simulink model "dynamic_QL"  (R2020b)
settings: Solver=VariableStepAuto  StartTime=0.0  StopTime=30.0  RelTol=1e-3
undefined symbols (not defined in the file or in its folder): loc, objects
libraries: mobileRoboticsLib x16, pid_lib x10
settings Model: Creator=Roozbeh  LastModifiedBy=Roozbeh

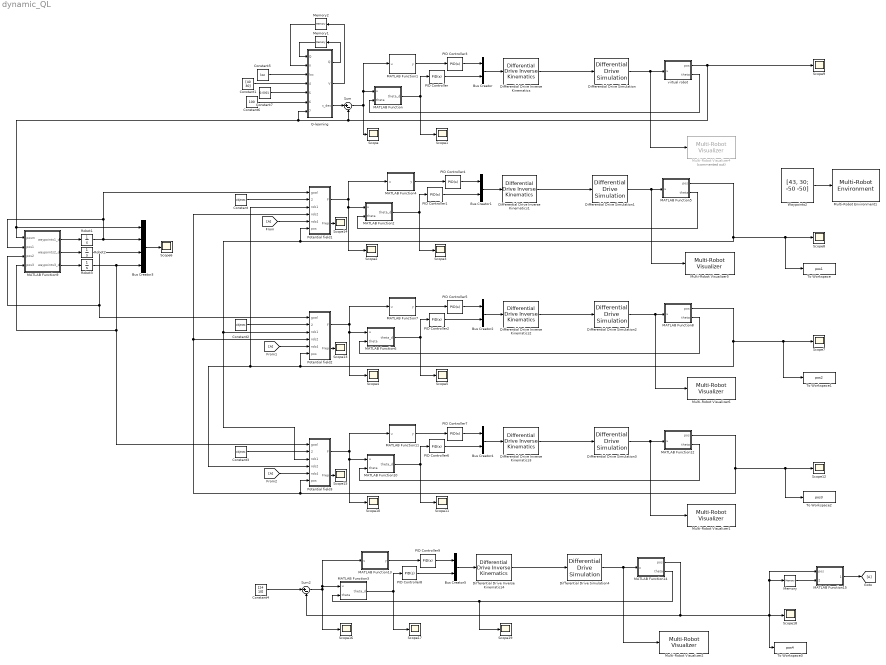
== system dynamic_QL ==
  Bus Creator{,1..2,4..5} (5 alike) : BusCreator  Inputs=2
  Bus Creator3 : BusCreator  Inputs=4
  Constant : Constant  Value=objects
  Constant1 : Constant  Value=[40 30]
  Constant2 : Constant  Value=objects
  Constant3 : Constant  Value=objects
  Constant4 : Constant  Value=[24 10]
  Constant5 : Constant  Value=loc
  Constant6 : Constant  Value=100
  Constant7 : Constant  Value=0.0001
  Differential Drive Inverse Kinematics{,1..4} (5 alike) : mobileRoboticsLib/Kinematic Models/Differential Drive/Differential Drive Inverse Kinematics  wheelRadius=0.1  wheelBase=0.5
      settings: SourceProductName=Mobile Robotics Simulation Toolbox
  Differential Drive Simulation : mobileRoboticsLib/Kinematic Models/Differential Drive/Differential Drive Simulation  wheelRadius=0.1  wheelBase=0.5  initX=6  initY=6  initAngle=0  Ts=0.05
      settings: SourceProductName=Mobile Robotics Simulation Toolbox
  Differential Drive Simulation1 : mobileRoboticsLib/Kinematic Models/Differential Drive/Differential Drive Simulation  wheelRadius=0.1  wheelBase=0.5  initX=8  initY=8  initAngle=0  Ts=0.05
      settings: SourceProductName=Mobile Robotics Simulation Toolbox
  Differential Drive Simulation2 : mobileRoboticsLib/Kinematic Models/Differential Drive/Differential Drive Simulation  wheelRadius=0.1  wheelBase=0.5  initX=4  initY=4  initAngle=0  Ts=0.05
      settings: SourceProductName=Mobile Robotics Simulation Toolbox
  Differential Drive Simulation3 : mobileRoboticsLib/Kinematic Models/Differential Drive/Differential Drive Simulation  wheelRadius=0.1  wheelBase=0.5  initX=4  initY=12  initAngle=0  Ts=0.05
      settings: SourceProductName=Mobile Robotics Simulation Toolbox
  Differential Drive Simulation4 : mobileRoboticsLib/Kinematic Models/Differential Drive/Differential Drive Simulation  wheelRadius=0.1  wheelBase=0.5  initX=24  initY=38  initAngle=0  Ts=0.05
      settings: SourceProductName=Mobile Robotics Simulation Toolbox
  MATLAB Function : MATLAB Function  TreatAsAtomicUnit=on
  MATLAB Function1 : MATLAB Function  TreatAsAtomicUnit=on
  MATLAB Function10 : MATLAB Function  TreatAsAtomicUnit=on
  MATLAB Function11 : MATLAB Function  TreatAsAtomicUnit=on
  MATLAB Function12 : MATLAB Function  TreatAsAtomicUnit=on
  MATLAB Function13 : MATLAB Function  TreatAsAtomicUnit=on
  MATLAB Function14 : MATLAB Function  TreatAsAtomicUnit=on
  MATLAB Function15 : MATLAB Function  TreatAsAtomicUnit=on
  MATLAB Function2 : MATLAB Function  TreatAsAtomicUnit=on
  MATLAB Function3 : MATLAB Function  TreatAsAtomicUnit=on
  MATLAB Function4 : MATLAB Function  TreatAsAtomicUnit=on
  MATLAB Function5 : MATLAB Function  TreatAsAtomicUnit=on
  MATLAB Function6 : MATLAB Function  TreatAsAtomicUnit=on
  MATLAB Function7 : MATLAB Function  TreatAsAtomicUnit=on
  MATLAB Function8 : MATLAB Function  TreatAsAtomicUnit=on
  MATLAB Function9 : MATLAB Function  TreatAsAtomicUnit=on
  Memory : Memory
  Memory1 : Memory  InitialCondition=zeros(size(loc,1) * size(loc,2), 8)
  Memory2 : Memory  InitialCondition=zeros(size(loc,1), size(loc,2))
  Multi-Robot Environment1 : mobileRoboticsLib/Environments/Multi-Robot Environment  numRobots=4  mapName=mapRooz  showWaypoints=on  showObjects=off  objectColors=[ 1, 0, 0; 0, 1, 0; 0, 0, 1 ]  objectMarkers='s'  showRobotIds=on  plotSensorLines=on
      settings: SourceProductName=Mobile Robotics Simulation Toolbox
  Multi-Robot Visualizer1 : mobileRoboticsLib/Environments/Multi-Robot Visualizer  idx=3  radius=0.5  robotColor=[0 0 1]  showTraj=off  hasLidar=off  sensorOffset=[0,0]  scanAngles=[-pi/4 0 pi/4]  maxNumScans=0  hasObjDetector=off  objDetectorOffset=[0,0]  objDetectorAngle=0  objDetectorFOV=pi/3  objDetectorMaxRange=5  hasRobotDetector=off  robotDetectorOffset=[0,0]  robotDetectorAngle=0  robotDetectorFOV=pi/3  robotDetectorMaxRange=5  robotDetectorNumDetections=0
      settings: SourceProductName=Mobile Robotics Simulation Toolbox
  Multi-Robot Visualizer2 : mobileRoboticsLib/Environments/Multi-Robot Visualizer  idx=4  radius=0.5  robotColor=[0 0 0]  showTraj=off  hasLidar=off  sensorOffset=[0,0]  scanAngles=[-pi/4 0 pi/4]  maxNumScans=0  hasObjDetector=off  objDetectorOffset=[0,0]  objDetectorAngle=0  objDetectorFOV=pi/3  objDetectorMaxRange=5  hasRobotDetector=off  robotDetectorOffset=[0,0]  robotDetectorAngle=0  robotDetectorFOV=pi/3  robotDetectorMaxRange=5  robotDetectorNumDetections=0
      settings: SourceProductName=Mobile Robotics Simulation Toolbox
  Multi-Robot Visualizer4 : mobileRoboticsLib/Environments/Multi-Robot Visualizer  Commented=on  idx=1  radius=0.5  robotColor=[0 0 1]  showTraj=off  hasLidar=off  sensorOffset=[0,0]  scanAngles=[-pi/4 0 pi/4]  maxNumScans=0  hasObjDetector=off  objDetectorOffset=[0,0]  objDetectorAngle=0  objDetectorFOV=pi/3  objDetectorMaxRange=5  hasRobotDetector=off  robotDetectorOffset=[0,0]  robotDetectorAngle=0  robotDetectorFOV=pi/3  robotDetectorMaxRange=5  robotDetectorNumDetections=0
      settings: SourceProductName=Mobile Robotics Simulation Toolbox
  Multi-Robot Visualizer5 : mobileRoboticsLib/Environments/Multi-Robot Visualizer  idx=1  radius=0.5  robotColor=[0 1 0]  showTraj=off  hasLidar=off  sensorOffset=[0,0]  scanAngles=[-pi/4 0 pi/4]  maxNumScans=0  hasObjDetector=off  objDetectorOffset=[0,0]  objDetectorAngle=0  objDetectorFOV=pi/3  objDetectorMaxRange=5  hasRobotDetector=off  robotDetectorOffset=[0,0]  robotDetectorAngle=0  robotDetectorFOV=pi/3  robotDetectorMaxRange=5  robotDetectorNumDetections=0
      settings: SourceProductName=Mobile Robotics Simulation Toolbox
  Multi-Robot Visualizer6 : mobileRoboticsLib/Environments/Multi-Robot Visualizer  idx=2  radius=0.5  robotColor=[1 0 0]  showTraj=off  hasLidar=off  sensorOffset=[0,0]  scanAngles=[-pi/4 0 pi/4]  maxNumScans=0  hasObjDetector=off  objDetectorOffset=[0,0]  objDetectorAngle=0  objDetectorFOV=pi/3  objDetectorMaxRange=5  hasRobotDetector=off  robotDetectorOffset=[0,0]  robotDetectorAngle=0  robotDetectorFOV=pi/3  robotDetectorMaxRange=5  robotDetectorNumDetections=0
      settings: SourceProductName=Mobile Robotics Simulation Toolbox
  PID Controller : pid_lib/PID Controller  Controller=PID  Form=Parallel  TimeDomain=Continuous-time  UseExternalTs=off  SampleTime=-1  IntegratorMethod=Forward Euler  FilterMethod=Forward Euler  ControllerParametersSource=internal  P=10  I=1  D=0  UseFilter=on  N=100  TunerSelectOption=Transfer Function Based (PID Tuner App)  InitialConditionSource=internal  InitialConditionForIntegrator=0  InitialConditionForFilter=0  DifferentiatorICPrevScaledInput=0  ExternalReset=none  TrackingMode=off  Kt=1  LimitOutput=off  SatLimitsSource=internal  UpperSaturationLimit=3  LowerSaturationLimit=-3  LinearizeAsGain=on  AntiWindupMode=none  Kb=1  POutMin=[]  POutMax=[]  IOutMin=[]  IOutMax=[]  DOutMin=[]  DOutMax=[]  NOutMin=[]  NOutMax=[]  SumOutMin=[]  SumOutMax=[]  SaturationOutMin=[]  SaturationOutMax=[]  PParamMin=[]  PParamMax=[]  IParamMin=[]  IParamMax=[]  DParamMin=[]  DParamMax=[]  NParamMin=[]  NParamMax=[]  KbParamMin=[]  KbParamMax=[]  KtParamMin=[]  KtParamMax=[]  KbOutMin=[]  KbOutMax=[]  KtOutMin=[]  KtOutMax=[]  IntegratorOutMin=[]  IntegratorOutMax=[]  FilterOutMin=[]  FilterOutMax=[]  SumI1OutMin=[]  SumI1OutMax=[]  SumI2OutMin=[]  SumI2OutMax=[]  SumI3OutMin=[]  SumI3OutMax=[]  SumI4OutMin=[]  SumI4OutMax=[]  SumDOutMin=[]  SumDOutMax=[]  DifferentiatorOutMin=[]  DifferentiatorOutMax=[]  FilterDiffOutCoefMin=[]  FilterDiffOutCoefMax=[]  ReciprocalOutMin=[]  ReciprocalOutMax=[]  SumDenOutMin=[]  SumDenOutMax=[]  SumNumOutMin=[]  SumNumOutMax=[]  DivideOutMin=[]  DivideOutMax=[]  UdiffTsProdOutMin=[]  UdiffTsProdOutMax=[]  NTsProdOutMin=[]  NTsProdOutMax=[]  UintegralTsProdOutMin=[]  UintegralTsProdOutMax=[]  UngainTsProdOutMin=[]  UngainTsProdOutMax=[]  IntegratorContinuousStateAttributes=''  IntegratorStateMustResolveToSignalObject=off  IntegratorRTWStateStorageClass=Auto  FilterContinuousStateAttributes=''  FilterStateMustResolveToSignalObject=off  FilterRTWStateStorageClass=Auto  ParallelPVariant=InternalParameters  IdealPVariant=Disabled  IVariant=InternalParameters  DVariant=InternalParameters  IntegratorVariant=Continuous  SatVariant=Disabled  AWVariant=Passthrough  PCopyVariant=Disabled  TRVariant=Disabled  FdbkBlocksVariant=Forward  IdealPFdbkVariant=Disabled  SatFdbkVariant=Disabled  DerivativeFilterVariant=ContFilter  NVariant=InternalParameters  NCopyVariant=Disabled  FilterICVariant=InternalICsFilter  IntegratorICVariant=InternalICs  ExternalResetVariant=Disabled  TRSumVariant=Passthrough  SumFdbkVariant=Disabled  SumVariant=Sum_PID  TsampFilterVariant=InternalTs  TsampNgainVariant=Passthrough  TsampIntegralVariant=Passthrough  ExternalSaturationOutDataTypeStr=Inherit: Same as second input
  PID Controller1 : pid_lib/PID Controller  Controller=PID  Form=Parallel  TimeDomain=Continuous-time  UseExternalTs=off  SampleTime=-1  IntegratorMethod=Forward Euler  FilterMethod=Forward Euler  ControllerParametersSource=internal  P=10  I=1  D=0  UseFilter=on  N=100  TunerSelectOption=Transfer Function Based (PID Tuner App)  InitialConditionSource=internal  InitialConditionForIntegrator=0  InitialConditionForFilter=0  DifferentiatorICPrevScaledInput=0  ExternalReset=none  TrackingMode=off  Kt=1  LimitOutput=on  SatLimitsSource=internal  UpperSaturationLimit=10  LowerSaturationLimit=-10  LinearizeAsGain=on  AntiWindupMode=none  Kb=1  POutMin=[]  POutMax=[]  IOutMin=[]  IOutMax=[]  DOutMin=[]  DOutMax=[]  NOutMin=[]  NOutMax=[]  SumOutMin=[]  SumOutMax=[]  SaturationOutMin=[]  SaturationOutMax=[]  PParamMin=[]  PParamMax=[]  IParamMin=[]  IParamMax=[]  DParamMin=[]  DParamMax=[]  NParamMin=[]  NParamMax=[]  KbParamMin=[]  KbParamMax=[]  KtParamMin=[]  KtParamMax=[]  KbOutMin=[]  KbOutMax=[]  KtOutMin=[]  KtOutMax=[]  IntegratorOutMin=[]  IntegratorOutMax=[]  FilterOutMin=[]  FilterOutMax=[]  SumI1OutMin=[]  SumI1OutMax=[]  SumI2OutMin=[]  SumI2OutMax=[]  SumI3OutMin=[]  SumI3OutMax=[]  SumI4OutMin=[]  SumI4OutMax=[]  SumDOutMin=[]  SumDOutMax=[]  DifferentiatorOutMin=[]  DifferentiatorOutMax=[]  FilterDiffOutCoefMin=[]  FilterDiffOutCoefMax=[]  ReciprocalOutMin=[]  ReciprocalOutMax=[]  SumDenOutMin=[]  SumDenOutMax=[]  SumNumOutMin=[]  SumNumOutMax=[]  DivideOutMin=[]  DivideOutMax=[]  UdiffTsProdOutMin=[]  UdiffTsProdOutMax=[]  NTsProdOutMin=[]  NTsProdOutMax=[]  UintegralTsProdOutMin=[]  UintegralTsProdOutMax=[]  UngainTsProdOutMin=[]  UngainTsProdOutMax=[]  IntegratorContinuousStateAttributes=''  IntegratorStateMustResolveToSignalObject=off  IntegratorRTWStateStorageClass=Auto  FilterContinuousStateAttributes=''  FilterStateMustResolveToSignalObject=off  FilterRTWStateStorageClass=Auto  ParallelPVariant=InternalParameters  IdealPVariant=Disabled  IVariant=InternalParameters  DVariant=InternalParameters  IntegratorVariant=Continuous  SatVariant=Enabled  AWVariant=Passthrough  PCopyVariant=Disabled  TRVariant=Disabled  FdbkBlocksVariant=Forward  IdealPFdbkVariant=Disabled  SatFdbkVariant=Disabled  DerivativeFilterVariant=ContFilter  NVariant=InternalParameters  NCopyVariant=Disabled  FilterICVariant=InternalICsFilter  IntegratorICVariant=InternalICs  ExternalResetVariant=Disabled  TRSumVariant=Passthrough  SumFdbkVariant=Disabled  SumVariant=Sum_PID  TsampFilterVariant=InternalTs  TsampNgainVariant=Passthrough  TsampIntegralVariant=Passthrough  ExternalSaturationOutDataTypeStr=Inherit: Same as second input
  PID Controller2 : pid_lib/PID Controller  Controller=PID  Form=Parallel  TimeDomain=Continuous-time  UseExternalTs=off  SampleTime=-1  IntegratorMethod=Forward Euler  FilterMethod=Forward Euler  ControllerParametersSource=internal  P=10  I=1  D=0  UseFilter=on  N=100  TunerSelectOption=Transfer Function Based (PID Tuner App)  InitialConditionSource=internal  InitialConditionForIntegrator=0  InitialConditionForFilter=0  DifferentiatorICPrevScaledInput=0  ExternalReset=none  TrackingMode=off  Kt=1  LimitOutput=on  SatLimitsSource=internal  UpperSaturationLimit=10  LowerSaturationLimit=-10  LinearizeAsGain=on  AntiWindupMode=none  Kb=1  POutMin=[]  POutMax=[]  IOutMin=[]  IOutMax=[]  DOutMin=[]  DOutMax=[]  NOutMin=[]  NOutMax=[]  SumOutMin=[]  SumOutMax=[]  SaturationOutMin=[]  SaturationOutMax=[]  PParamMin=[]  PParamMax=[]  IParamMin=[]  IParamMax=[]  DParamMin=[]  DParamMax=[]  NParamMin=[]  NParamMax=[]  KbParamMin=[]  KbParamMax=[]  KtParamMin=[]  KtParamMax=[]  KbOutMin=[]  KbOutMax=[]  KtOutMin=[]  KtOutMax=[]  IntegratorOutMin=[]  IntegratorOutMax=[]  FilterOutMin=[]  FilterOutMax=[]  SumI1OutMin=[]  SumI1OutMax=[]  SumI2OutMin=[]  SumI2OutMax=[]  SumI3OutMin=[]  SumI3OutMax=[]  SumI4OutMin=[]  SumI4OutMax=[]  SumDOutMin=[]  SumDOutMax=[]  DifferentiatorOutMin=[]  DifferentiatorOutMax=[]  FilterDiffOutCoefMin=[]  FilterDiffOutCoefMax=[]  ReciprocalOutMin=[]  ReciprocalOutMax=[]  SumDenOutMin=[]  SumDenOutMax=[]  SumNumOutMin=[]  SumNumOutMax=[]  DivideOutMin=[]  DivideOutMax=[]  UdiffTsProdOutMin=[]  UdiffTsProdOutMax=[]  NTsProdOutMin=[]  NTsProdOutMax=[]  UintegralTsProdOutMin=[]  UintegralTsProdOutMax=[]  UngainTsProdOutMin=[]  UngainTsProdOutMax=[]  IntegratorContinuousStateAttributes=''  IntegratorStateMustResolveToSignalObject=off  IntegratorRTWStateStorageClass=Auto  FilterContinuousStateAttributes=''  FilterStateMustResolveToSignalObject=off  FilterRTWStateStorageClass=Auto  ParallelPVariant=InternalParameters  IdealPVariant=Disabled  IVariant=InternalParameters  DVariant=InternalParameters  IntegratorVariant=Continuous  SatVariant=Enabled  AWVariant=Passthrough  PCopyVariant=Disabled  TRVariant=Disabled  FdbkBlocksVariant=Forward  IdealPFdbkVariant=Disabled  SatFdbkVariant=Disabled  DerivativeFilterVariant=ContFilter  NVariant=InternalParameters  NCopyVariant=Disabled  FilterICVariant=InternalICsFilter  IntegratorICVariant=InternalICs  ExternalResetVariant=Disabled  TRSumVariant=Passthrough  SumFdbkVariant=Disabled  SumVariant=Sum_PID  TsampFilterVariant=InternalTs  TsampNgainVariant=Passthrough  TsampIntegralVariant=Passthrough  ExternalSaturationOutDataTypeStr=Inherit: Same as second input
  PID Controller3 : pid_lib/PID Controller  Controller=PID  Form=Parallel  TimeDomain=Continuous-time  UseExternalTs=off  SampleTime=-1  IntegratorMethod=Forward Euler  FilterMethod=Forward Euler  ControllerParametersSource=internal  P=5  I=0  D=0.1  UseFilter=on  N=100  TunerSelectOption=Transfer Function Based (PID Tuner App)  InitialConditionSource=internal  InitialConditionForIntegrator=0  InitialConditionForFilter=0  DifferentiatorICPrevScaledInput=0  ExternalReset=none  TrackingMode=off  Kt=1  LimitOutput=on  SatLimitsSource=internal  UpperSaturationLimit=3  LowerSaturationLimit=-3  LinearizeAsGain=on  AntiWindupMode=none  Kb=1  POutMin=[]  POutMax=[]  IOutMin=[]  IOutMax=[]  DOutMin=[]  DOutMax=[]  NOutMin=[]  NOutMax=[]  SumOutMin=[]  SumOutMax=[]  SaturationOutMin=[]  SaturationOutMax=[]  PParamMin=[]  PParamMax=[]  IParamMin=[]  IParamMax=[]  DParamMin=[]  DParamMax=[]  NParamMin=[]  NParamMax=[]  KbParamMin=[]  KbParamMax=[]  KtParamMin=[]  KtParamMax=[]  KbOutMin=[]  KbOutMax=[]  KtOutMin=[]  KtOutMax=[]  IntegratorOutMin=[]  IntegratorOutMax=[]  FilterOutMin=[]  FilterOutMax=[]  SumI1OutMin=[]  SumI1OutMax=[]  SumI2OutMin=[]  SumI2OutMax=[]  SumI3OutMin=[]  SumI3OutMax=[]  SumI4OutMin=[]  SumI4OutMax=[]  SumDOutMin=[]  SumDOutMax=[]  DifferentiatorOutMin=[]  DifferentiatorOutMax=[]  FilterDiffOutCoefMin=[]  FilterDiffOutCoefMax=[]  ReciprocalOutMin=[]  ReciprocalOutMax=[]  SumDenOutMin=[]  SumDenOutMax=[]  SumNumOutMin=[]  SumNumOutMax=[]  DivideOutMin=[]  DivideOutMax=[]  UdiffTsProdOutMin=[]  UdiffTsProdOutMax=[]  NTsProdOutMin=[]  NTsProdOutMax=[]  UintegralTsProdOutMin=[]  UintegralTsProdOutMax=[]  UngainTsProdOutMin=[]  UngainTsProdOutMax=[]  IntegratorContinuousStateAttributes=''  IntegratorStateMustResolveToSignalObject=off  IntegratorRTWStateStorageClass=Auto  FilterContinuousStateAttributes=''  FilterStateMustResolveToSignalObject=off  FilterRTWStateStorageClass=Auto  ParallelPVariant=InternalParameters  IdealPVariant=Disabled  IVariant=InternalParameters  DVariant=InternalParameters  IntegratorVariant=Continuous  SatVariant=Enabled  AWVariant=Passthrough  PCopyVariant=Disabled  TRVariant=Disabled  FdbkBlocksVariant=Forward  IdealPFdbkVariant=Disabled  SatFdbkVariant=Disabled  DerivativeFilterVariant=ContFilter  NVariant=InternalParameters  NCopyVariant=Disabled  FilterICVariant=InternalICsFilter  IntegratorICVariant=InternalICs  ExternalResetVariant=Disabled  TRSumVariant=Passthrough  SumFdbkVariant=Disabled  SumVariant=Sum_PID  TsampFilterVariant=InternalTs  TsampNgainVariant=Passthrough  TsampIntegralVariant=Passthrough  ExternalSaturationOutDataTypeStr=Inherit: Same as second input
  PID Controller4 : pid_lib/PID Controller  Controller=PID  Form=Parallel  TimeDomain=Continuous-time  UseExternalTs=off  SampleTime=-1  IntegratorMethod=Forward Euler  FilterMethod=Forward Euler  ControllerParametersSource=internal  P=5  I=0  D=0.1  UseFilter=on  N=100  TunerSelectOption=Transfer Function Based (PID Tuner App)  InitialConditionSource=internal  InitialConditionForIntegrator=0  InitialConditionForFilter=0  DifferentiatorICPrevScaledInput=0  ExternalReset=none  TrackingMode=off  Kt=1  LimitOutput=on  SatLimitsSource=internal  UpperSaturationLimit=5  LowerSaturationLimit=-5  LinearizeAsGain=on  AntiWindupMode=none  Kb=1  POutMin=[]  POutMax=[]  IOutMin=[]  IOutMax=[]  DOutMin=[]  DOutMax=[]  NOutMin=[]  NOutMax=[]  SumOutMin=[]  SumOutMax=[]  SaturationOutMin=[]  SaturationOutMax=[]  PParamMin=[]  PParamMax=[]  IParamMin=[]  IParamMax=[]  DParamMin=[]  DParamMax=[]  NParamMin=[]  NParamMax=[]  KbParamMin=[]  KbParamMax=[]  KtParamMin=[]  KtParamMax=[]  KbOutMin=[]  KbOutMax=[]  KtOutMin=[]  KtOutMax=[]  IntegratorOutMin=[]  IntegratorOutMax=[]  FilterOutMin=[]  FilterOutMax=[]  SumI1OutMin=[]  SumI1OutMax=[]  SumI2OutMin=[]  SumI2OutMax=[]  SumI3OutMin=[]  SumI3OutMax=[]  SumI4OutMin=[]  SumI4OutMax=[]  SumDOutMin=[]  SumDOutMax=[]  DifferentiatorOutMin=[]  DifferentiatorOutMax=[]  FilterDiffOutCoefMin=[]  FilterDiffOutCoefMax=[]  ReciprocalOutMin=[]  ReciprocalOutMax=[]  SumDenOutMin=[]  SumDenOutMax=[]  SumNumOutMin=[]  SumNumOutMax=[]  DivideOutMin=[]  DivideOutMax=[]  UdiffTsProdOutMin=[]  UdiffTsProdOutMax=[]  NTsProdOutMin=[]  NTsProdOutMax=[]  UintegralTsProdOutMin=[]  UintegralTsProdOutMax=[]  UngainTsProdOutMin=[]  UngainTsProdOutMax=[]  IntegratorContinuousStateAttributes=''  IntegratorStateMustResolveToSignalObject=off  IntegratorRTWStateStorageClass=Auto  FilterContinuousStateAttributes=''  FilterStateMustResolveToSignalObject=off  FilterRTWStateStorageClass=Auto  ParallelPVariant=InternalParameters  IdealPVariant=Disabled  IVariant=InternalParameters  DVariant=InternalParameters  IntegratorVariant=Continuous  SatVariant=Enabled  AWVariant=Passthrough  PCopyVariant=Disabled  TRVariant=Disabled  FdbkBlocksVariant=Forward  IdealPFdbkVariant=Disabled  SatFdbkVariant=Disabled  DerivativeFilterVariant=ContFilter  NVariant=InternalParameters  NCopyVariant=Disabled  FilterICVariant=InternalICsFilter  IntegratorICVariant=InternalICs  ExternalResetVariant=Disabled  TRSumVariant=Passthrough  SumFdbkVariant=Disabled  SumVariant=Sum_PID  TsampFilterVariant=InternalTs  TsampNgainVariant=Passthrough  TsampIntegralVariant=Passthrough  ExternalSaturationOutDataTypeStr=Inherit: Same as second input
  PID Controller5 : pid_lib/PID Controller  Controller=PID  Form=Parallel  TimeDomain=Continuous-time  UseExternalTs=off  SampleTime=-1  IntegratorMethod=Forward Euler  FilterMethod=Forward Euler  ControllerParametersSource=internal  P=5  I=0  D=0.1  UseFilter=on  N=100  TunerSelectOption=Transfer Function Based (PID Tuner App)  InitialConditionSource=internal  InitialConditionForIntegrator=0  InitialConditionForFilter=0  DifferentiatorICPrevScaledInput=0  ExternalReset=none  TrackingMode=off  Kt=1  LimitOutput=on  SatLimitsSource=internal  UpperSaturationLimit=5  LowerSaturationLimit=-5  LinearizeAsGain=on  AntiWindupMode=none  Kb=1  POutMin=[]  POutMax=[]  IOutMin=[]  IOutMax=[]  DOutMin=[]  DOutMax=[]  NOutMin=[]  NOutMax=[]  SumOutMin=[]  SumOutMax=[]  SaturationOutMin=[]  SaturationOutMax=[]  PParamMin=[]  PParamMax=[]  IParamMin=[]  IParamMax=[]  DParamMin=[]  DParamMax=[]  NParamMin=[]  NParamMax=[]  KbParamMin=[]  KbParamMax=[]  KtParamMin=[]  KtParamMax=[]  KbOutMin=[]  KbOutMax=[]  KtOutMin=[]  KtOutMax=[]  IntegratorOutMin=[]  IntegratorOutMax=[]  FilterOutMin=[]  FilterOutMax=[]  SumI1OutMin=[]  SumI1OutMax=[]  SumI2OutMin=[]  SumI2OutMax=[]  SumI3OutMin=[]  SumI3OutMax=[]  SumI4OutMin=[]  SumI4OutMax=[]  SumDOutMin=[]  SumDOutMax=[]  DifferentiatorOutMin=[]  DifferentiatorOutMax=[]  FilterDiffOutCoefMin=[]  FilterDiffOutCoefMax=[]  ReciprocalOutMin=[]  ReciprocalOutMax=[]  SumDenOutMin=[]  SumDenOutMax=[]  SumNumOutMin=[]  SumNumOutMax=[]  DivideOutMin=[]  DivideOutMax=[]  UdiffTsProdOutMin=[]  UdiffTsProdOutMax=[]  NTsProdOutMin=[]  NTsProdOutMax=[]  UintegralTsProdOutMin=[]  UintegralTsProdOutMax=[]  UngainTsProdOutMin=[]  UngainTsProdOutMax=[]  IntegratorContinuousStateAttributes=''  IntegratorStateMustResolveToSignalObject=off  IntegratorRTWStateStorageClass=Auto  FilterContinuousStateAttributes=''  FilterStateMustResolveToSignalObject=off  FilterRTWStateStorageClass=Auto  ParallelPVariant=InternalParameters  IdealPVariant=Disabled  IVariant=InternalParameters  DVariant=InternalParameters  IntegratorVariant=Continuous  SatVariant=Enabled  AWVariant=Passthrough  PCopyVariant=Disabled  TRVariant=Disabled  FdbkBlocksVariant=Forward  IdealPFdbkVariant=Disabled  SatFdbkVariant=Disabled  DerivativeFilterVariant=ContFilter  NVariant=InternalParameters  NCopyVariant=Disabled  FilterICVariant=InternalICsFilter  IntegratorICVariant=InternalICs  ExternalResetVariant=Disabled  TRSumVariant=Passthrough  SumFdbkVariant=Disabled  SumVariant=Sum_PID  TsampFilterVariant=InternalTs  TsampNgainVariant=Passthrough  TsampIntegralVariant=Passthrough  ExternalSaturationOutDataTypeStr=Inherit: Same as second input
  PID Controller6 : pid_lib/PID Controller  Controller=PID  Form=Parallel  TimeDomain=Continuous-time  UseExternalTs=off  SampleTime=-1  IntegratorMethod=Forward Euler  FilterMethod=Forward Euler  ControllerParametersSource=internal  P=10  I=1  D=0  UseFilter=on  N=100  TunerSelectOption=Transfer Function Based (PID Tuner App)  InitialConditionSource=internal  InitialConditionForIntegrator=0  InitialConditionForFilter=0  DifferentiatorICPrevScaledInput=0  ExternalReset=none  TrackingMode=off  Kt=1  LimitOutput=on  SatLimitsSource=internal  UpperSaturationLimit=10  LowerSaturationLimit=-10  LinearizeAsGain=on  AntiWindupMode=none  Kb=1  POutMin=[]  POutMax=[]  IOutMin=[]  IOutMax=[]  DOutMin=[]  DOutMax=[]  NOutMin=[]  NOutMax=[]  SumOutMin=[]  SumOutMax=[]  SaturationOutMin=[]  SaturationOutMax=[]  PParamMin=[]  PParamMax=[]  IParamMin=[]  IParamMax=[]  DParamMin=[]  DParamMax=[]  NParamMin=[]  NParamMax=[]  KbParamMin=[]  KbParamMax=[]  KtParamMin=[]  KtParamMax=[]  KbOutMin=[]  KbOutMax=[]  KtOutMin=[]  KtOutMax=[]  IntegratorOutMin=[]  IntegratorOutMax=[]  FilterOutMin=[]  FilterOutMax=[]  SumI1OutMin=[]  SumI1OutMax=[]  SumI2OutMin=[]  SumI2OutMax=[]  SumI3OutMin=[]  SumI3OutMax=[]  SumI4OutMin=[]  SumI4OutMax=[]  SumDOutMin=[]  SumDOutMax=[]  DifferentiatorOutMin=[]  DifferentiatorOutMax=[]  FilterDiffOutCoefMin=[]  FilterDiffOutCoefMax=[]  ReciprocalOutMin=[]  ReciprocalOutMax=[]  SumDenOutMin=[]  SumDenOutMax=[]  SumNumOutMin=[]  SumNumOutMax=[]  DivideOutMin=[]  DivideOutMax=[]  UdiffTsProdOutMin=[]  UdiffTsProdOutMax=[]  NTsProdOutMin=[]  NTsProdOutMax=[]  UintegralTsProdOutMin=[]  UintegralTsProdOutMax=[]  UngainTsProdOutMin=[]  UngainTsProdOutMax=[]  IntegratorContinuousStateAttributes=''  IntegratorStateMustResolveToSignalObject=off  IntegratorRTWStateStorageClass=Auto  FilterContinuousStateAttributes=''  FilterStateMustResolveToSignalObject=off  FilterRTWStateStorageClass=Auto  ParallelPVariant=InternalParameters  IdealPVariant=Disabled  IVariant=InternalParameters  DVariant=InternalParameters  IntegratorVariant=Continuous  SatVariant=Enabled  AWVariant=Passthrough  PCopyVariant=Disabled  TRVariant=Disabled  FdbkBlocksVariant=Forward  IdealPFdbkVariant=Disabled  SatFdbkVariant=Disabled  DerivativeFilterVariant=ContFilter  NVariant=InternalParameters  NCopyVariant=Disabled  FilterICVariant=InternalICsFilter  IntegratorICVariant=InternalICs  ExternalResetVariant=Disabled  TRSumVariant=Passthrough  SumFdbkVariant=Disabled  SumVariant=Sum_PID  TsampFilterVariant=InternalTs  TsampNgainVariant=Passthrough  TsampIntegralVariant=Passthrough  ExternalSaturationOutDataTypeStr=Inherit: Same as second input
  PID Controller7 : pid_lib/PID Controller  Controller=PID  Form=Parallel  TimeDomain=Continuous-time  UseExternalTs=off  SampleTime=-1  IntegratorMethod=Forward Euler  FilterMethod=Forward Euler  ControllerParametersSource=internal  P=5  I=0  D=0.1  UseFilter=on  N=100  TunerSelectOption=Transfer Function Based (PID Tuner App)  InitialConditionSource=internal  InitialConditionForIntegrator=0  InitialConditionForFilter=0  DifferentiatorICPrevScaledInput=0  ExternalReset=none  TrackingMode=off  Kt=1  LimitOutput=on  SatLimitsSource=internal  UpperSaturationLimit=5  LowerSaturationLimit=-5  LinearizeAsGain=on  AntiWindupMode=none  Kb=1  POutMin=[]  POutMax=[]  IOutMin=[]  IOutMax=[]  DOutMin=[]  DOutMax=[]  NOutMin=[]  NOutMax=[]  SumOutMin=[]  SumOutMax=[]  SaturationOutMin=[]  SaturationOutMax=[]  PParamMin=[]  PParamMax=[]  IParamMin=[]  IParamMax=[]  DParamMin=[]  DParamMax=[]  NParamMin=[]  NParamMax=[]  KbParamMin=[]  KbParamMax=[]  KtParamMin=[]  KtParamMax=[]  KbOutMin=[]  KbOutMax=[]  KtOutMin=[]  KtOutMax=[]  IntegratorOutMin=[]  IntegratorOutMax=[]  FilterOutMin=[]  FilterOutMax=[]  SumI1OutMin=[]  SumI1OutMax=[]  SumI2OutMin=[]  SumI2OutMax=[]  SumI3OutMin=[]  SumI3OutMax=[]  SumI4OutMin=[]  SumI4OutMax=[]  SumDOutMin=[]  SumDOutMax=[]  DifferentiatorOutMin=[]  DifferentiatorOutMax=[]  FilterDiffOutCoefMin=[]  FilterDiffOutCoefMax=[]  ReciprocalOutMin=[]  ReciprocalOutMax=[]  SumDenOutMin=[]  SumDenOutMax=[]  SumNumOutMin=[]  SumNumOutMax=[]  DivideOutMin=[]  DivideOutMax=[]  UdiffTsProdOutMin=[]  UdiffTsProdOutMax=[]  NTsProdOutMin=[]  NTsProdOutMax=[]  UintegralTsProdOutMin=[]  UintegralTsProdOutMax=[]  UngainTsProdOutMin=[]  UngainTsProdOutMax=[]  IntegratorContinuousStateAttributes=''  IntegratorStateMustResolveToSignalObject=off  IntegratorRTWStateStorageClass=Auto  FilterContinuousStateAttributes=''  FilterStateMustResolveToSignalObject=off  FilterRTWStateStorageClass=Auto  ParallelPVariant=InternalParameters  IdealPVariant=Disabled  IVariant=InternalParameters  DVariant=InternalParameters  IntegratorVariant=Continuous  SatVariant=Enabled  AWVariant=Passthrough  PCopyVariant=Disabled  TRVariant=Disabled  FdbkBlocksVariant=Forward  IdealPFdbkVariant=Disabled  SatFdbkVariant=Disabled  DerivativeFilterVariant=ContFilter  NVariant=InternalParameters  NCopyVariant=Disabled  FilterICVariant=InternalICsFilter  IntegratorICVariant=InternalICs  ExternalResetVariant=Disabled  TRSumVariant=Passthrough  SumFdbkVariant=Disabled  SumVariant=Sum_PID  TsampFilterVariant=InternalTs  TsampNgainVariant=Passthrough  TsampIntegralVariant=Passthrough  ExternalSaturationOutDataTypeStr=Inherit: Same as second input
  PID Controller8 : pid_lib/PID Controller  Controller=PID  Form=Parallel  TimeDomain=Continuous-time  UseExternalTs=off  SampleTime=-1  IntegratorMethod=Forward Euler  FilterMethod=Forward Euler  ControllerParametersSource=internal  P=10  I=0  D=0  UseFilter=on  N=100  TunerSelectOption=Transfer Function Based (PID Tuner App)  InitialConditionSource=internal  InitialConditionForIntegrator=0  InitialConditionForFilter=0  DifferentiatorICPrevScaledInput=0  ExternalReset=none  TrackingMode=off  Kt=1  LimitOutput=off  SatLimitsSource=internal  UpperSaturationLimit=inf  LowerSaturationLimit=-inf  LinearizeAsGain=on  AntiWindupMode=none  Kb=1  POutMin=[]  POutMax=[]  IOutMin=[]  IOutMax=[]  DOutMin=[]  DOutMax=[]  NOutMin=[]  NOutMax=[]  SumOutMin=[]  SumOutMax=[]  SaturationOutMin=[]  SaturationOutMax=[]  PParamMin=[]  PParamMax=[]  IParamMin=[]  IParamMax=[]  DParamMin=[]  DParamMax=[]  NParamMin=[]  NParamMax=[]  KbParamMin=[]  KbParamMax=[]  KtParamMin=[]  KtParamMax=[]  KbOutMin=[]  KbOutMax=[]  KtOutMin=[]  KtOutMax=[]  IntegratorOutMin=[]  IntegratorOutMax=[]  FilterOutMin=[]  FilterOutMax=[]  SumI1OutMin=[]  SumI1OutMax=[]  SumI2OutMin=[]  SumI2OutMax=[]  SumI3OutMin=[]  SumI3OutMax=[]  SumI4OutMin=[]  SumI4OutMax=[]  SumDOutMin=[]  SumDOutMax=[]  DifferentiatorOutMin=[]  DifferentiatorOutMax=[]  FilterDiffOutCoefMin=[]  FilterDiffOutCoefMax=[]  ReciprocalOutMin=[]  ReciprocalOutMax=[]  SumDenOutMin=[]  SumDenOutMax=[]  SumNumOutMin=[]  SumNumOutMax=[]  DivideOutMin=[]  DivideOutMax=[]  UdiffTsProdOutMin=[]  UdiffTsProdOutMax=[]  NTsProdOutMin=[]  NTsProdOutMax=[]  UintegralTsProdOutMin=[]  UintegralTsProdOutMax=[]  UngainTsProdOutMin=[]  UngainTsProdOutMax=[]  IntegratorContinuousStateAttributes=''  IntegratorStateMustResolveToSignalObject=off  IntegratorRTWStateStorageClass=Auto  FilterContinuousStateAttributes=''  FilterStateMustResolveToSignalObject=off  FilterRTWStateStorageClass=Auto  ParallelPVariant=InternalParameters  IdealPVariant=Disabled  IVariant=InternalParameters  DVariant=InternalParameters  IntegratorVariant=Continuous  SatVariant=Disabled  AWVariant=Passthrough  PCopyVariant=Disabled  TRVariant=Disabled  FdbkBlocksVariant=Forward  IdealPFdbkVariant=Disabled  SatFdbkVariant=Disabled  DerivativeFilterVariant=ContFilter  NVariant=InternalParameters  NCopyVariant=Disabled  FilterICVariant=InternalICsFilter  IntegratorICVariant=InternalICs  ExternalResetVariant=Disabled  TRSumVariant=Passthrough  SumFdbkVariant=Disabled  SumVariant=Sum_PID  TsampFilterVariant=InternalTs  TsampNgainVariant=Passthrough  TsampIntegralVariant=Passthrough  ExternalSaturationOutDataTypeStr=Inherit: Same as second input
  PID Controller9 : pid_lib/PID Controller  Controller=PID  Form=Parallel  TimeDomain=Continuous-time  UseExternalTs=off  SampleTime=-1  IntegratorMethod=Forward Euler  FilterMethod=Forward Euler  ControllerParametersSource=internal  P=1  I=0  D=0  UseFilter=on  N=100  TunerSelectOption=Transfer Function Based (PID Tuner App)  InitialConditionSource=internal  InitialConditionForIntegrator=0  InitialConditionForFilter=0  DifferentiatorICPrevScaledInput=0  ExternalReset=none  TrackingMode=off  Kt=1  LimitOutput=on  SatLimitsSource=internal  UpperSaturationLimit=1.8  LowerSaturationLimit=-1.8  LinearizeAsGain=on  AntiWindupMode=none  Kb=1  POutMin=[]  POutMax=[]  IOutMin=[]  IOutMax=[]  DOutMin=[]  DOutMax=[]  NOutMin=[]  NOutMax=[]  SumOutMin=[]  SumOutMax=[]  SaturationOutMin=[]  SaturationOutMax=[]  PParamMin=[]  PParamMax=[]  IParamMin=[]  IParamMax=[]  DParamMin=[]  DParamMax=[]  NParamMin=[]  NParamMax=[]  KbParamMin=[]  KbParamMax=[]  KtParamMin=[]  KtParamMax=[]  KbOutMin=[]  KbOutMax=[]  KtOutMin=[]  KtOutMax=[]  IntegratorOutMin=[]  IntegratorOutMax=[]  FilterOutMin=[]  FilterOutMax=[]  SumI1OutMin=[]  SumI1OutMax=[]  SumI2OutMin=[]  SumI2OutMax=[]  SumI3OutMin=[]  SumI3OutMax=[]  SumI4OutMin=[]  SumI4OutMax=[]  SumDOutMin=[]  SumDOutMax=[]  DifferentiatorOutMin=[]  DifferentiatorOutMax=[]  FilterDiffOutCoefMin=[]  FilterDiffOutCoefMax=[]  ReciprocalOutMin=[]  ReciprocalOutMax=[]  SumDenOutMin=[]  SumDenOutMax=[]  SumNumOutMin=[]  SumNumOutMax=[]  DivideOutMin=[]  DivideOutMax=[]  UdiffTsProdOutMin=[]  UdiffTsProdOutMax=[]  NTsProdOutMin=[]  NTsProdOutMax=[]  UintegralTsProdOutMin=[]  UintegralTsProdOutMax=[]  UngainTsProdOutMin=[]  UngainTsProdOutMax=[]  IntegratorContinuousStateAttributes=''  IntegratorStateMustResolveToSignalObject=off  IntegratorRTWStateStorageClass=Auto  FilterContinuousStateAttributes=''  FilterStateMustResolveToSignalObject=off  FilterRTWStateStorageClass=Auto  ParallelPVariant=InternalParameters  IdealPVariant=Disabled  IVariant=InternalParameters  DVariant=InternalParameters  IntegratorVariant=Continuous  SatVariant=Enabled  AWVariant=Passthrough  PCopyVariant=Disabled  TRVariant=Disabled  FdbkBlocksVariant=Forward  IdealPFdbkVariant=Disabled  SatFdbkVariant=Disabled  DerivativeFilterVariant=ContFilter  NVariant=InternalParameters  NCopyVariant=Disabled  FilterICVariant=InternalICsFilter  IntegratorICVariant=InternalICs  ExternalResetVariant=Disabled  TRSumVariant=Passthrough  SumFdbkVariant=Disabled  SumVariant=Sum_PID  TsampFilterVariant=InternalTs  TsampNgainVariant=Passthrough  TsampIntegralVariant=Passthrough  ExternalSaturationOutDataTypeStr=Inherit: Same as second input
  Potential field1 : MATLAB Function  TreatAsAtomicUnit=on
  Potential field2 : MATLAB Function  TreatAsAtomicUnit=on
  Potential field3 : MATLAB Function  TreatAsAtomicUnit=on
  Q-learning : MATLAB Function  TreatAsAtomicUnit=on
  Robot1 : Integrator  InitialCondition=[8 8]
  Robot2 : Integrator  InitialCondition=[4 5]
  Robot3 : Integrator  InitialCondition=[4 11]
  Scope{,1..19} (20 alike) : Scope
  Sum : Sum  Inputs=|+-
  Sum2 : Sum  Inputs=|+-
  To Workspace : ToWorkspace  VariableName=pos1  SaveFormat=Timeseries  SampleTime=-1
  To Workspace1 : ToWorkspace  VariableName=pos2  SaveFormat=Timeseries  SampleTime=-1
  To Workspace2 : ToWorkspace  VariableName=pos3  SaveFormat=Timeseries  SampleTime=-1
  To Workspace3 : ToWorkspace  VariableName=pos4  SaveFormat=Timeseries  SampleTime=-1
  Waypoints2 : Constant  Value=[43, 30; -50 -50]
  virtual robot : MATLAB Function  TreatAsAtomicUnit=on
  wires:
  [A] -> Potential field1/5(rob4)
  [A] -> Potential field3/5(rob4)
  Differential Drive Inverse Kinematics1/1 -> Differential Drive Simulation1/1
  MATLAB Function1/1(y) -> PID Controller3/1
  Robot1/1 -> Potential field1/1(goal), MATLAB Function9/2(pos1), Bus Creator3/2
  virtual robot/2(theta) -> MATLAB Function/2(theta)
  MATLAB Function15/1(pos_future) -> [A]
  Potential field1/1(F) -> Scope2/1, MATLAB Function2/1(u), MATLAB Function4/1(u)
  [A] -> Potential field2/5(rob4)
  MATLAB Function6/1(theta_d) -> PID Controller2/1, Scope5/1
  Differential Drive Simulation2/1 -> Multi-Robot Visualizer6/1, MATLAB Function8/1(u)
  MATLAB Function2/1(theta_d) -> PID Controller1/1, Scope3/1
  MATLAB Function12/1(pos) -> To Workspace2/1, Scope12/1, Potential field1/4(rob2), Potential field2/4(rob2), Potential field3/6(pos)
  MATLAB Function8/1(pos) -> To Workspace1/1, Scope7/1, Potential field3/4(rob2), Potential field1/3(rob1), Potential field2/6(pos)
  PID Controller5/1 -> Bus Creator2/1
  Waypoints2/1 -> Multi-Robot Environment1/1
  Differential Drive Simulation4/1 -> MATLAB Function14/1(u), Multi-Robot Visualizer2/1
  virtual robot/1(pos) -> MATLAB Function9/1(posm), Bus Creator3/1, Q-learning/7(start_state), Sum/2, Scope9/1
  MATLAB Function9/2(waypoints2_d) -> Robot2/1
  Differential Drive Inverse Kinematics2/1 -> Differential Drive Simulation2/1
  MATLAB Function10/1(theta_d) -> PID Controller6/1, Scope11/1
  Constant5/1 -> Q-learning/3(loc)
  Constant/1 -> Potential field1/2(objects)
  MATLAB Function9/3(waypoints3_d) -> Robot3/1
  Differential Drive Simulation1/1 -> Multi-Robot Visualizer5/1, MATLAB Function5/1(u)
  Bus Creator4/1 -> Differential Drive Inverse Kinematics3/1
  MATLAB Function7/1(y) -> PID Controller5/1
  Robot3/1 -> MATLAB Function9/4(pos3), Potential field3/1(goal), Bus Creator3/4
  MATLAB Function3/1(theta_d) -> PID Controller8/1, Scope17/1
  Bus Creator2/1 -> Differential Drive Inverse Kinematics2/1
  Potential field3/2(Frep) -> Scope15/1
  Potential field2/1(F) -> Scope4/1, MATLAB Function6/1(u), MATLAB Function7/1(u)
  PID Controller4/1 -> Bus Creator1/1
  PID Controller2/1 -> Bus Creator2/2
  Memory/1 -> MATLAB Function15/2(pos_old)
  Bus Creator3/1 -> Scope6/1
  Differential Drive Simulation/1 -> Multi-Robot Visualizer4/1, virtual robot/1(u)
  MATLAB Function11/1(y) -> PID Controller7/1
  PID Controller6/1 -> Bus Creator4/2
  Potential field1/2(Frep) -> Scope14/1
  PID Controller7/1 -> Bus Creator4/1
  MATLAB Function9/1(waypoints1_d) -> Robot1/1
  Bus Creator/1 -> Differential Drive Inverse Kinematics/1
  Potential field2/2(Frep) -> Scope13/1
  Sum/1 -> MATLAB Function1/1(u), MATLAB Function/1(u), Scope/1
  MATLAB Function8/2(theta) -> MATLAB Function6/2(theta)
  Bus Creator5/1 -> Differential Drive Inverse Kinematics4/1
  PID Controller3/1 -> Bus Creator/1
  Constant2/1 -> Potential field2/2(objects)
  MATLAB Function/1(theta_d) -> PID Controller/1, Scope1/1
  Constant3/1 -> Potential field3/2(objects)
  MATLAB Function5/1(pos) -> To Workspace/1, Scope8/1, Potential field1/6(pos), Potential field3/3(rob1), Potential field2/3(rob1)
  MATLAB Function12/2(theta) -> MATLAB Function10/2(theta)
  Differential Drive Inverse Kinematics3/1 -> Differential Drive Simulation3/1
  PID Controller8/1 -> Bus Creator5/2
  Robot2/1 -> MATLAB Function9/3(pos2), Potential field2/1(goal), Bus Creator3/3
  Constant4/1 -> Sum2/1
  MATLAB Function4/1(y) -> PID Controller4/1
  MATLAB Function5/2(theta) -> MATLAB Function2/2(theta)
  PID Controller9/1 -> Bus Creator5/1
  PID Controller/1 -> Bus Creator/2
  Differential Drive Inverse Kinematics/1 -> Differential Drive Simulation/1
  Differential Drive Simulation3/1 -> Multi-Robot Visualizer1/1, MATLAB Function12/1(u)
  Sum2/1 -> MATLAB Function3/1(u), MATLAB Function13/1(u), Scope16/1
  Differential Drive Inverse Kinematics4/1 -> Differential Drive Simulation4/1
  Bus Creator1/1 -> Differential Drive Inverse Kinematics1/1
  Constant1/1 -> Q-learning/4(goal_state)
  MATLAB Function14/1(pos) -> Sum2/2, Memory/1, MATLAB Function15/1(pos), To Workspace3/1, Scope18/1
  Potential field3/1(F) -> Scope10/1, MATLAB Function10/1(u), MATLAB Function11/1(u)
  MATLAB Function14/2(theta) -> MATLAB Function3/2(theta), Scope19/1
  PID Controller1/1 -> Bus Creator1/2
  MATLAB Function13/1(y) -> PID Controller9/1
  Q-learning/3(x_des) -> Sum/1
  Constant6/1 -> Q-learning/6(maxIter)
  Constant7/1 -> Q-learning/5(stop_rate)
  Q-learning/1(Q) -> Memory1/1
  Memory1/1 -> Q-learning/1("Q ")
  Q-learning/2(V) -> Memory2/1
  Memory2/1 -> Q-learning/2("V ")

== matlab function dynamic_QL/MATLAB Function8 ==
  data: u input; pos output; theta output
function [pos, theta] = fcn(u)

pos = u(1:2);
theta = u(3);

== matlab function dynamic_QL/MATLAB Function9 ==
  data: posm input; waypoints1_d output; pos1 input; waypoints2_d output; pos2 input; pos3 input; waypoints3_d output
function [waypoints1_d, waypoints2_d, waypoints3_d] = fcn(posm, pos1, pos2, pos3)

L = [-3 1 1 1; 1 -3 1 1; 1 1 -3 1; 1 1 1 -3];
F = [-3 0; 0 0; -4 -3; -4 3];
x = [posm(1:2)'; pos1(1:2)'; pos2(1:2)'; pos3(1:2)'];
xd = L*(x - F);

waypoints1_d = xd(2,:);
waypoints2_d = xd(3,:);
waypoints3_d = xd(4,:);

== matlab function dynamic_QL/MATLAB Function10 ==
  data: u input; theta_d output; theta input
function theta_d = fcn(u, theta)

delta = atan2(u(2), u(1)) - theta;
sgn = sign(delta);
delta_hat = delta - 2*pi*sgn;
if abs(delta_hat) < abs(delta)
    theta_d = delta_hat;
else
    theta_d = delta;
end

== matlab function dynamic_QL/MATLAB Function11 ==
  data: u input; y output
function y = fcn(u)

y = sqrt(u(1)^2 + u(2)^2);

== matlab function dynamic_QL/MATLAB Function12 ==
  data: u input; pos output; theta output
function [pos, theta] = fcn(u)

pos = u(1:2);
theta = u(3);

== matlab function dynamic_QL/Potential field1 ==
  data: goal input; objects input; rob1 input; rob2 input; rob4 input; pos input; F output; Frep output
function [F, Frep]  = fcn(goal, objects, rob1, rob2, rob4, pos)
% initialization - user variables
zeta = 1;
d = 3;
etha = 20;
ro = 4;

objects = [objects; rob1'; rob2'; rob4'];

% att
dist = pos - goal;
dist_norm = norm(dist);
if dist_norm > d
    Fatt = -d*zeta*dist/dist_norm;
else
    Fatt = -zeta*dist;
end

% repel
Frep = [0; 0];
for i = 1:1:size(objects,1)
    dist_obj = objects(i,:)' - pos;
    dist_obj_norm = norm(dist_obj);
    if dist_obj_norm < ro
        Frep = Frep + etha*(1/dist_obj_norm - 1/ro) * dist_obj / (dist_obj_norm^3);
    end
end

% total
F = Fatt - Frep;

== matlab function dynamic_QL/Potential field2 ==
  data: goal input; objects input; rob1 input; rob2 input; rob4 input; pos input; F output; Frep output
function [F, Frep]  = fcn(goal, objects, rob1, rob2, rob4, pos)
% initialization - user variables
zeta = 1;
d = 3;
etha = 20;
ro = 4;

objects = [objects; rob1'; rob2'; rob4'];

% att
dist = pos - goal;
dist_norm = norm(dist);
if dist_norm > d
    Fatt = -d*zeta*dist/dist_norm;
else
    Fatt = -zeta*dist;
end

% repel
Frep = [0; 0];
for i = 1:1:size(objects,1)
    dist_obj = objects(i,:)' - pos;
    dist_obj_norm = norm(dist_obj);
    if dist_obj_norm < ro
        Frep = Frep + etha*(1/dist_obj_norm - 1/ro) * dist_obj / (dist_obj_norm^3);
    end
end

% total
F = Fatt - Frep;

== matlab function dynamic_QL/Potential field3 ==
  data: goal input; objects input; rob1 input; rob2 input; rob4 input; pos input; F output; Frep output
function [F, Frep]  = fcn(goal, objects, rob1, rob2, rob4, pos)
% initialization - user variables
zeta = 1;
d = 3;
etha = 20;
ro = 4;

objects = [objects; rob1'; rob2'; rob4'];

% att
dist = pos - goal;
dist_norm = norm(dist);
if dist_norm > d
    Fatt = -d*zeta*dist/dist_norm;
else
    Fatt = -zeta*dist;
end

% repel
Frep = [0; 0];
for i = 1:1:size(objects,1)
    dist_obj = objects(i,:)' - pos;
    dist_obj_norm = norm(dist_obj);
    if dist_obj_norm < ro
        Frep = Frep + etha*(1/dist_obj_norm - 1/ro) * dist_obj / (dist_obj_norm^3);
    end
end

% total
F = Fatt - Frep;

== matlab function dynamic_QL/MATLAB Function13 ==
  data: u input; y output
function y = fcn(u)

y = sqrt(u(1)^2 + u(2)^2);

== matlab function dynamic_QL/MATLAB Function14 ==
  data: u input; pos output; theta output
function [pos, theta] = fcn(u)

pos = u(1:2);
theta = u(3);

== matlab function dynamic_QL/MATLAB Function3 ==
  data: u input; theta_d output; theta input
function theta_d = fcn(u, theta)

delta = atan2(u(2), u(1)) - theta;
sgn = sign(delta);
delta_hat = delta - 2*pi*sgn;
if abs(delta_hat) < abs(delta)
    theta_d = delta_hat;
else
    theta_d = delta;
end

== matlab function dynamic_QL/MATLAB Function15 ==
  data: pos input; pos_future output; pos_old input
function pos_future = fcn(pos, pos_old)

v = pos - pos_old;
pos_future = pos + v;

== matlab function dynamic_QL/MATLAB Function ==
  data: u input; theta_d output; theta input
function theta_d = fcn(u, theta)

delta = atan2(u(2), u(1)) - theta;
sgn = sign(delta);
delta_hat = delta - 2*pi*sgn;
if abs(delta_hat) < abs(delta)
    theta_d = delta_hat;
else
    theta_d = delta;
end

== matlab function dynamic_QL/Q-learning ==
  data: Q input; V input; loc input; goal_state input; stop_rate input; maxIter input; start_state input; Q output; V output; x_des output
function [Q, V, x_des] = Q_learning_p(Q, V, loc, goal_state, stop_rate, maxIter, start_state)
% parameters
alpha = 0.9;
gama = 0.9;

% Actions = {N, S, E, W, NW, NE, SW, SE} |A| = 8
actions = [0 1; 0 -1; 1 0; -1 0; -1 1; 1 1; -1 -1; 1 -1]; % direction of Actions in x-y coordination
numActions = size(actions,1);
m = size(loc,1);
n = size(loc,2);
Pi = ones(m*n, numActions) / numActions;
iter = 0;
while iter < maxIter
    delta = 0;
    for x = 1:m
        for y = 1:n
            s = (y-1)*m + x;
            v = V(x,y);
            for a = 1:numActions
                pos = [x y] + actions(a,:);
                %R = -norm(pos - goal_state)/1000 + norm([x y] - goal_state)/1000;
                %R = -1;
                R = -norm(actions(a,:));
                %R = -norm(pos - goal_state)/1000;
                if pos(1) < 1 || pos(1) > m || pos(2) < 1 || pos(2) > n || loc(round(pos(1)), round(pos(2))) == 1
                    Q(s,a) = -10;
                else
                    if pos(1) == goal_state(1) && pos(2) == goal_state(2)
                        R = 10;
                    end
                    Q(s,a) = (1-alpha)*Q(s,a) + alpha*(R + gama*V(pos(1), pos(2)));
                end
            end
            V(x,y) = max(Q(s,:));
            delta = max(delta, abs(v-V(x,y)));
            Pi(s,:) = Q(s,:) - min(Q(s,:));
            Pi(s,:) = Pi(s,:) / sum(Pi(s,:));
        end
    end
  
    if delta < stop_rate
        break
    end
    iter = iter + 1;
    
end

[~, I] = max(Pi,[],2,'linear');
policy = ceil(I/(m*n));
policy = reshape(policy, m, n);

s = round(start_state');
if s(1) == goal_state(1) && s(2) == goal_state(2)
    x_des = s;
else
    x_des = s + actions(policy(s(1),s(2)),:);
end

== matlab function dynamic_QL/MATLAB Function1 ==
  data: u input; y output
function y = fcn(u)

y = 0.5*sqrt(u(1)^2 + u(2)^2);

== matlab function dynamic_QL/virtual robot ==
  data: u input; pos output; theta output
function [pos, theta] = fcn(u)

pos = u(1:2);
theta = u(3);

== matlab function dynamic_QL/MATLAB Function2 ==
  data: u input; theta_d output; theta input
function theta_d = fcn(u, theta)

delta = atan2(u(2), u(1)) - theta;
sgn = sign(delta);
delta_hat = delta - 2*pi*sgn;
if abs(delta_hat) < abs(delta)
    theta_d = delta_hat;
else
    theta_d = delta;
end

== matlab function dynamic_QL/MATLAB Function4 ==
  data: u input; y output
function y = fcn(u)

y = sqrt(u(1)^2 + u(2)^2);

== matlab function dynamic_QL/MATLAB Function5 ==
  data: u input; pos output; theta output
function [pos, theta] = fcn(u)

pos = u(1:2);
theta = u(3);

== matlab function dynamic_QL/MATLAB Function6 ==
  data: u input; theta_d output; theta input
function theta_d = fcn(u, theta)

delta = atan2(u(2), u(1)) - theta;
sgn = sign(delta);
delta_hat = delta - 2*pi*sgn;
if abs(delta_hat) < abs(delta)
    theta_d = delta_hat;
else
    theta_d = delta;
end

== matlab function dynamic_QL/MATLAB Function7 ==
  data: u input; y output
function y = fcn(u)

y = sqrt(u(1)^2 + u(2)^2);
